simulink model "drone_interface"  (R2018b)
settings: Solver=VariableStepAuto  StartTime=0.0  StopTime=10.0  RelTol=1e-3
settings Model: Creator=Alistair  LastModifiedBy=Alistair

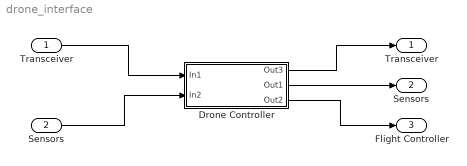
== system drone_interface ==
  Transceiver : Inport
  Sensors : Inport  Port=2
  Drone Controller : Subsystem
  "Transceiver " : Outport
  "Sensors " : Outport  Port=2
  Flight Controller : Outport  Port=3
  wires:
  Drone Controller/2(Out1) -> "Sensors "/1
  Drone Controller/1(Out3) -> "Transceiver "/1
  Drone Controller/3(Out2) -> Flight Controller/1
  Transceiver/1 -> Drone Controller/1(In1)
  Sensors/1 -> Drone Controller/2(In2)

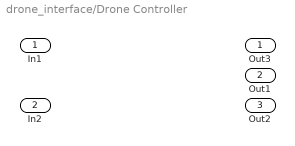
== system drone_interface/Drone Controller ==
  In1 : Inport
  In2 : Inport  Port=2
  Out3 : Outport
  Out1 : Outport  Port=2
  Out2 : Outport  Port=3
